simulink model "Respiratory"  (Simulink 6.4)
settings: Solver=ode45  StartTime=0.0  StopTime=10.0  RelTol=1e-3
values from neighbouring files (symbols this model uses):
  a1 = 0.3836    [Dissociation_Spencer_IC.m]    (also in Gas_Exchange_IC.m; Respiratory_IC.m)
  a2 = 1.819    [Dissociation_Spencer_IC.m]    (also in Gas_Exchange_IC.m; Respiratory_IC.m)
  alpha1 = 0.02598    [Dissociation_Spencer_IC.m]    (also in Gas_Exchange_IC.m; Respiratory_IC.m)
  alpha2 = 0.05591    [Dissociation_Spencer_IC.m]    (also in Gas_Exchange_IC.m; Respiratory_IC.m)
  beta1 = 0.012275    [Dissociation_Spencer_IC.m]    (also in Gas_Exchange_IC.m; Respiratory_IC.m)
  beta2 = 0.03255    [Dissociation_Spencer_IC.m]    (also in Gas_Exchange_IC.m; Respiratory_IC.m)
  C1 = 9    [Dissociation_Spencer_IC.m]    (also in Gas_Exchange_IC.m; Respiratory_IC.m)
  C2 = 87.00    (= 87)    [Dissociation_Spencer_IC.m]    (also in Gas_Exchange_IC.m; Respiratory_IC.m)
  Circadian_Period = 24    [Respiratory_IC.m]    (also in State_UA_Khoo_IC.m)
  CvCO2IC = 0.5116    [Body_Khoo_IC.m]    (also in Gas_Exchange_IC.m; Respiratory_IC.m = 0.5247)
  CvO2IC = 0.1672    [Body_Khoo_IC.m]    (also in Gas_Exchange_IC.m; Respiratory_IC.m = 0.1639)
  Dead1CO2IC = 0.1020    (= 0.102)    [Dead_Space_Khoo_IC.m]    (also in Gas_Exchange_IC.m; Respiratory_IC.m = 39.5616)
  Dead1O2IC = 149.8824    [Dead_Space_Khoo_IC.m]    (also in Gas_Exchange_IC.m; Respiratory_IC.m = 104.3637)
  Dead2CO2IC = 0.5274    [Dead_Space_Khoo_IC.m]    (also in Gas_Exchange_IC.m; Respiratory_IC.m = 39.6736)
  Dead2O2IC = 149.3923    [Dead_Space_Khoo_IC.m]    (also in Gas_Exchange_IC.m; Respiratory_IC.m = 104.2258)
  Dead3CO2IC = 2.2996    [Dead_Space_Khoo_IC.m]    (also in Gas_Exchange_IC.m; Respiratory_IC.m = 39.8127)
  Dead3O2IC = 147.3503    [Dead_Space_Khoo_IC.m]    (also in Gas_Exchange_IC.m; Respiratory_IC.m = 104.0505)
  Dead4CO2IC = 8.2293    [Dead_Space_Khoo_IC.m]    (also in Gas_Exchange_IC.m; Respiratory_IC.m = 40.0061)
  Dead4O2IC = 140.5179    [Dead_Space_Khoo_IC.m]    (also in Gas_Exchange_IC.m; Respiratory_IC.m = 103.8005)
  Dead5CO2IC = 22.0757    [Dead_Space_Khoo_IC.m]    (also in Gas_Exchange_IC.m; Respiratory_IC.m = 40.3359)
  Dead5O2IC = 124.5641    [Dead_Space_Khoo_IC.m]    (also in Gas_Exchange_IC.m; Respiratory_IC.m = 103.3579)
  E_CW = 5    [Pleural_Schuessler_IC.m]    (also in Pmus_Flow_Younes_IC.m; Resp_Mech_IC.m; Respiratory_IC.m)
  E_L = 5    [Pleural_Schuessler_IC.m]    (also in Pmus_Flow_Younes_IC.m; Resp_Mech_IC.m; Respiratory_IC.m)
  fc = 0.4/60    (= 0.00666666666667)    [Respiratory_IC.m]    (also in State_UA_Khoo_IC.m)
  FlowIC = 0    [Pmus_Flow_Younes_IC.m]    (also in Resp_Mech_IC.m; Respiratory_IC.m)
  gc = 0.008/60    (= 0.000133333333333)    [Respiratory_IC.m]    (also in State_UA_Khoo_IC.m)
  h = 0.0183    [Brain_Khoo_IC.m]    (also in Gas_Exchange_IC.m; Respiratory_IC.m)
  K1 = 13    [Dissociation_Spencer_IC.m]    (also in Gas_Exchange_IC.m; Respiratory_IC.m)
  K2 = 194.4    [Dissociation_Spencer_IC.m]    (also in Gas_Exchange_IC.m; Respiratory_IC.m)
  MRbCO2 = 0.0517    [Brain_Khoo_IC.m]    (also in Gas_Exchange_IC.m; Respiratory_IC.m)
  MRCO2 = 0.0033    [Body_Khoo_IC.m]    (also in Gas_Exchange_IC.m; Respiratory_IC.m)
  MRO2 = 0.0038    [Body_Khoo_IC.m]    (also in Gas_Exchange_IC.m; Respiratory_IC.m)
  PACO2_delayIC = 39.6041    [Cardio_Mix_Lange_IC.m]    (also in Gas_Exchange_IC.m; Respiratory_IC.m = 40.4448)
  PaCO2firstIC = 0.2150    (= 0.215)    [Cardio_Mix_Lange_IC.m]    (also in Gas_Exchange_IC.m; Respiratory_IC.m = -0.2465)
  PACO2IC = 37.1484    [Gas_Exchange_IC.m]    (also in Lungs_Khoo_IC.m; Respiratory_IC.m = 40.9432)
  PaCO2secondIC = 38.4577    [Cardio_Mix_Lange_IC.m]    (also in Gas_Exchange_IC.m; Respiratory_IC.m = 40.3928)
  PAO2_delayIC = 103.8436    [Cardio_Mix_Lange_IC.m]    (also in Gas_Exchange_IC.m; Respiratory_IC.m = 103.1223)
  PaO2firstIC = -0.2838    [Cardio_Mix_Lange_IC.m]    (also in Gas_Exchange_IC.m; Respiratory_IC.m = 0.3557)
  PAO2IC = 107.1983    [Gas_Exchange_IC.m]    (also in Lungs_Khoo_IC.m; Respiratory_IC.m = 102.5153)
  PaO2secondIC = 105.4828    [Cardio_Mix_Lange_IC.m]    (also in Gas_Exchange_IC.m; Respiratory_IC.m = 103.1435)
  PbCO2IC = 48.2858    [Brain_Khoo_IC.m]    (also in Gas_Exchange_IC.m; Respiratory_IC.m = 48.5383)
  PICO2 = 0    [Dead_Space_Khoo_IC.m]    (also in Gas_Exchange_IC.m; Respiratory_IC.m)
  PICO2_change = 0    [Respiratory_IC.m]
  PIO2 = 150    [Dead_Space_Khoo_IC.m]    (also in Gas_Exchange_IC.m; Respiratory_IC.m)
  PIO2_change = -90    [Mech_vent_test.m]    (also in Respiratory_IC.m = 0)
  Pt_frcIC1 = 0    [Pmus_Flow_Younes_IC.m]    (also in Resp_Mech_IC.m; Respiratory_IC.m)
  Pt_frcIC2 = 0    [Pmus_Flow_Younes_IC.m]    (also in Resp_Mech_IC.m; Respiratory_IC.m)
  QdBo = 0.8333    [Brain_Khoo_IC.m]    (also in Gas_Exchange_IC.m; Respiratory_IC.m)
  R_AW = 1.27    [Pleural_Schuessler_IC.m]    (also in Pmus_Flow_Younes_IC.m; Resp_Mech_IC.m; Respiratory_IC.m)
  R_CW = 1.03    [Pleural_Schuessler_IC.m]    (also in Pmus_Flow_Younes_IC.m; Resp_Mech_IC.m; Respiratory_IC.m)
  R_L = 1.69    [Pleural_Schuessler_IC.m]    (also in Pmus_Flow_Younes_IC.m; Resp_Mech_IC.m; Respiratory_IC.m)
  RC = 0.06    [Pleural_Schuessler_IC.m]    (also in Pmus_Flow_Younes_IC.m; Resp_Mech_IC.m; Respiratory_IC.m)
  rc = 0.2/60    (= 0.00333333333333)    [Respiratory_IC.m]    (also in State_UA_Khoo_IC.m)
  SbCO2 = 0.3600    (= 0.36)    [Brain_Khoo_IC.m]    (also in Gas_Exchange_IC.m; Respiratory_IC.m)
  SCO2 = 0.0043    [Brain_Khoo_IC.m]    (also in Gas_Exchange_IC.m; Respiratory_IC.m)
  SWAo = 0.007    [Respiratory_IC.m]    (also in State_UA_Khoo_IC.m)
  T1 = 1    [Cardio_Mix_Lange_IC.m]    (also in Gas_Exchange_IC.m; Respiratory_IC.m)
  T2 = 2    [Cardio_Mix_Lange_IC.m]    (also in Gas_Exchange_IC.m; Respiratory_IC.m)
  t_CO2_duration = 0    [Respiratory_IC.m]
  t_CO2_start = 0    [Respiratory_IC.m]
  t_end_UA = 0    [Respiratory_IC.m]    (also in State_UA_Khoo_IC.m)
  t_O2_duration = 0    [Mech_vent_test.m]    (also in Respiratory_IC.m)
  t_O2_start = 0    [Mech_vent_test.m]    (also in Respiratory_IC.m)
  t_start_UA = 0    [Respiratory_IC.m]    (also in State_UA_Khoo_IC.m)
  time_step = time_step    [acquire_data.m]    (also in acquire_data_save.m)
  VC = 5    [Pmus_Flow_Younes_IC.m]    (also in Resp_Mech_IC.m; Respiratory_IC.m)
  Vdead1 = 0.03    [Dead_Space_Khoo_IC.m]    (also in Gas_Exchange_IC.m; Respiratory_IC.m)
  Vdead2 = 0.03    [Dead_Space_Khoo_IC.m]    (also in Gas_Exchange_IC.m; Respiratory_IC.m)
  Vdead3 = 0.03    [Dead_Space_Khoo_IC.m]    (also in Gas_Exchange_IC.m; Respiratory_IC.m)
  Vdead4 = 0.03    [Dead_Space_Khoo_IC.m]    (also in Gas_Exchange_IC.m; Respiratory_IC.m)
  Vdead5 = 0.03    [Dead_Space_Khoo_IC.m]    (also in Gas_Exchange_IC.m; Respiratory_IC.m)
  VTCO2 = 15    [Body_Khoo_IC.m]    (also in Gas_Exchange_IC.m; Respiratory_IC.m)
  VtIC = 0    [Pmus_Flow_Younes_IC.m]    (also in Resp_Mech_IC.m; Respiratory_IC.m)
  VTO2 = 6    [Body_Khoo_IC.m]    (also in Gas_Exchange_IC.m; Respiratory_IC.m)
  Z = 0.0227    [Dissociation_Spencer_IC.m]    (also in Gas_Exchange_IC.m; Respiratory_IC.m)
undefined symbols (not defined in the file or in its folder): A_0_ua, Arousal_UAIC, b_ua, C_ua_awake, DAY, K_ua, R_LAW, R_trachea
libraries: simulink x1, simulink_extras x1
(part 2 of 2)

== system Respiratory/Gas Exchange/GAS EXCHANGE IN THE LUNGS/CO2 Gas Exchange in the Lungs ==
  CaCO2 : Inport
  CVCO2 : Inport  Port=2
  Pd5CO2 : Inport  Port=3
  Vt - Tidal Volume : Inport  Port=4
  Flow : Inport  Port=5
  "Q " : Inport  Port=6
  Fcn -11 blocks : Fcn  Expr=(((u(2) >=0) * u(2) * u(1) + (u(2) <0) * 0 ) + (u(3) - u(4)) *u(5) * ( lambda*(1-s) ) )/( u(6)+VLCO2 )
  Integrator : Integrator  InitialCondition=PACO2IC
  Mux : Mux  Inputs=6
  sum1 : Sum  Inputs=-+  SaturateOnIntegerOverflow=on  InputSameDT=on
  PACO2 : Outport
  tag scope: PACO2IC=global
  wires:
  "Q "/1 -> Mux/5
  CVCO2/1 -> Mux/3
  CaCO2/1 -> Mux/4
  Fcn -11 blocks/1 -> Integrator/1
  Integrator/1 -> [PACO2IC], PACO2/1, sum1/1
  Pd5CO2/1 -> sum1/2
  Mux/1 -> Fcn -11 blocks/1
  sum1/1 -> Mux/1
  Flow/1 -> Mux/2
  Vt - Tidal Volume/1 -> Mux/6

== system Respiratory/Gas Exchange/GAS EXCHANGE IN THE LUNGS/O2 Gas Exchange in the Lungs ==
  Vt - Tidal Volume : Inport
  Flow : Inport  Port=2
  Q : Inport  Port=3
  CaO2 : Inport  Port=4
  CVO2 : Inport  Port=5
  Pd5O2 : Inport  Port=6
  Fcn -11 blocks : Fcn  Expr=(((u(2) >=0) * u(2) * u(1) + (u(2) <0) * 0 ) + (u(4) - u(5)) *u(3) * ( lambda*(1-s) ) )/( u(6)+VLO2 )
  Integrator : Integrator  InitialCondition=PAO2IC  LimitOutput=on  LowerSaturationLimit=0
  Mux : Mux  Inputs=6
  Sum2 : Sum  Inputs=-+  SaturateOnIntegerOverflow=on  InputSameDT=on
  PAO2 : Outport
  tag scope: PAO2IC=global
  wires:
  Integrator/1 -> PAO2/1, [PAO2IC], Sum2/1
  Fcn -11 blocks/1 -> Integrator/1
  Pd5O2/1 -> Sum2/2
  Mux/1 -> Fcn -11 blocks/1
  Sum2/1 -> Mux/1
  Flow/1 -> Mux/2
  Q/1 -> Mux/3
  CVO2/1 -> Mux/4
  CaO2/1 -> Mux/5
  Vt - Tidal Volume/1 -> Mux/6

== system Respiratory/Respiratory_Mechanics/Pleural_Pressure1/Pa ==
  "Flow   " : Inport
  "Pao " : Inport  Port=2
  Fcn : Fcn  Expr=(u>=0)*u * (kaw1 + abs( (u>=0)*u) *kaw2)
  Fcn1 : Fcn  Expr=(u>=0)*u
  Sum2 : Sum  Inputs=+-  SaturateOnIntegerOverflow=on  InputSameDT=on
  "Pa " : Outport
  wires:
  "Flow   "/1 -> Fcn/1
  "Pao "/1 -> Sum2/1
  Sum2/1 -> Fcn1/1
  Fcn/1 -> Sum2/2
  Fcn1/1 -> "Pa "/1

== system Respiratory/Respiratory_Mechanics/Pleural_Pressure1/Pcw ==
  Vt : Inport
  Flow : Inport  Port=2
  Fcn : Fcn  Expr=(u>=0)*u
  Pcw_0 : Constant  Value=-1  OutDataType=sfix(16)  ConRadixGroup=Use specified scaling  OutScaling=2^0  SampleTime=inf  FramePeriod=inf
  Product3 : Product  SaturateOnIntegerOverflow=on  InputSameDT=on
  Product4 : Product  SaturateOnIntegerOverflow=on  InputSameDT=on
  Sum3 : Sum  Inputs=+++  SaturateOnIntegerOverflow=on  InputSameDT=on
  elastance : Constant  Value=E_CW  OutDataType=sfix(16)  ConRadixGroup=Use specified scaling  OutScaling=2^0  SampleTime=inf  FramePeriod=inf
  "resistance " : Constant  Value=R_CW  OutDataType=sfix(16)  ConRadixGroup=Use specified scaling  OutScaling=2^0  SampleTime=inf  FramePeriod=inf
  "Pcw  " : Outport
  wires:
  Fcn/1 -> Product3/2
  Vt/1 -> Product4/1
  elastance/1 -> Product4/2
  Sum3/1 -> "Pcw  "/1
  Product4/1 -> Sum3/2
  Flow/1 -> Fcn/1
  Product3/1 -> Sum3/1
  "resistance "/1 -> Product3/1
  Pcw_0/1 -> Sum3/3

== system Respiratory/Respiratory_Mechanics/Respiratory Muscles Activity1/Resp Muscle Reaction ==
  RespMus Drive : Inport
  Step Size : Inport  Port=2
  0.735539 : Gain
  Fcn : Fcn  Expr=u(1) + u(2) + (u(2) *u(5)/u(4) - u(3)+u(1)) * (exp(-u(4)/u(5)) - 1)
  Memory : Memory  X0=Pt_frcIC1  InheritSampleTime=on
  Memory1 : Memory  Orientation=left  X0=Pt_frcIC2  InheritSampleTime=on  LinearizeMemory=on
  Mux : Mux  Inputs=5
  RC1 : Constant  Value=RC  OutDataType=sfix(16)  ConRadixGroup=Use specified scaling  OutScaling=2^0  SampleTime=inf  FramePeriod=inf
  Sum4 : Sum  Inputs=+-  SaturateOnIntegerOverflow=on  InputSameDT=on
  Pt_frc : Outport
  wires:
  RespMus Drive/1 -> Sum4/1, Memory/1
  Sum4/1 -> Mux/2
  RC1/1 -> Mux/5
  Step Size/1 -> Mux/4
  Memory1/1 -> Mux/1
  Memory/1 -> Sum4/2, Mux/3
  Mux/1 -> Fcn/1
  Fcn/1 -> 0.735539/1
  0.735539/1 -> Pt_frc/1, Memory1/1

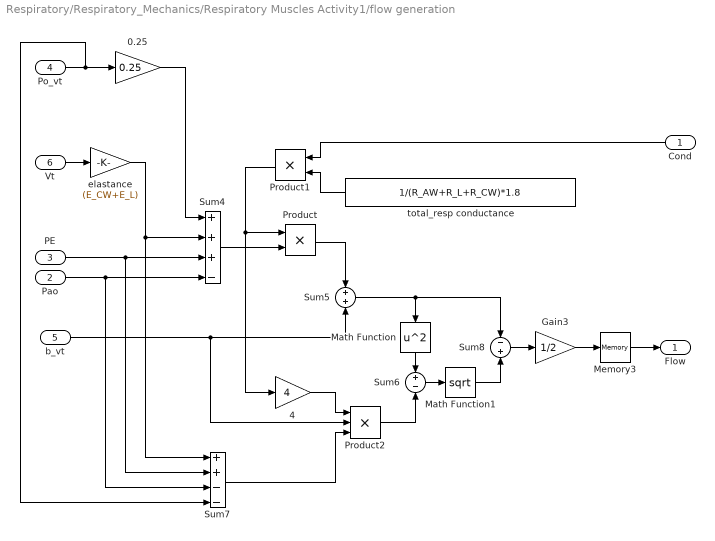
== system Respiratory/Respiratory_Mechanics/Respiratory Muscles Activity1/flow generation ==
  "Cond " : Inport  Orientation=left
  "Pao " : Inport  Port=2
  PE : Inport  Port=3
  "Po_vt " : Inport  Port=4
  b_vt : Inport  Port=5
  Vt : Inport  Port=6
  0.25 : Gain  Gain=0.25  SaturateOnIntegerOverflow=on
  4 : Gain  Gain=4  SaturateOnIntegerOverflow=on
  Gain3 : Gain  Gain=1/2  SaturateOnIntegerOverflow=on
  Math Function : Math  Orientation=down  Operator=square  SaturateOnIntegerOverflow=on
  Math Function1 : Math  Operator=sqrt  SaturateOnIntegerOverflow=on
  Memory3 : Memory  X0=FlowIC  InheritSampleTime=on
  Product : Product  SaturateOnIntegerOverflow=on  InputSameDT=on
  Product1 : Product  Orientation=left  SaturateOnIntegerOverflow=on  InputSameDT=on
  Product2 : Product  Inputs=3  SaturateOnIntegerOverflow=on  InputSameDT=on
  Sum4 : Sum  Inputs=+++-  SaturateOnIntegerOverflow=on  InputSameDT=on
  Sum5 : Sum  SaturateOnIntegerOverflow=on  InputSameDT=on
  Sum6 : Sum  Inputs=+-  SaturateOnIntegerOverflow=on  InputSameDT=on
  Sum7 : Sum  Inputs=++--  SaturateOnIntegerOverflow=on  InputSameDT=on
  Sum8 : Sum  Inputs=-+  SaturateOnIntegerOverflow=on  InputSameDT=on
  elastance : Gain  Gain=(E_CW+E_L)  SaturateOnIntegerOverflow=on
  total_resp conductance : Constant  Orientation=left  Value=1/(R_AW+R_L+R_CW)*1.8  OutDataType=sfix(16)  ConRadixGroup=Use specified scaling  OutScaling=2^0  SampleTime=inf  FramePeriod=inf
  Flow : Outport
  wires:
  0.25/1 -> Sum4/1
  total_resp conductance/1 -> Product1/2
  "Cond "/1 -> Product1/1
  Product1/1 -> 4/1, Product/1
  Gain3/1 -> Memory3/1
  Sum8/1 -> Gain3/1
  Sum5/1 -> Sum8/1, Math Function/1
  Math Function1/1 -> Sum8/2
  Sum6/1 -> Math Function1/1
  Product2/1 -> Sum6/2
  "Po_vt "/1 -> Sum7/4, 0.25/1
  "Pao "/1 -> Sum7/3, Sum4/4
  PE/1 -> Sum7/2, Sum4/3
  elastance/1 -> Sum7/1, Sum4/2
  Sum7/1 -> Product2/3
  b_vt/1 -> Product2/2, Sum5/2
  4/1 -> Product2/1
  Math Function/1 -> Sum6/1
  Product/1 -> Sum5/1
  Sum4/1 -> Product/2
  Vt/1 -> elastance/1
  Memory3/1 -> Flow/1

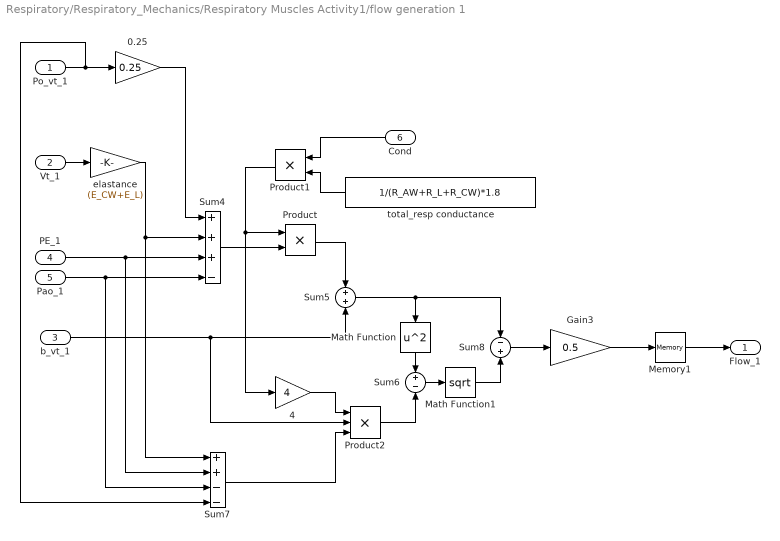
== system Respiratory/Respiratory_Mechanics/Respiratory Muscles Activity1/flow generation 1 ==
  Po_vt_1 : Inport
  Vt_1 : Inport  Port=2
  b_vt_1 : Inport  Port=3
  PE_1 : Inport  Port=4
  Pao_1 : Inport  Port=5
  "Cond " : Inport  Orientation=left  Port=6
  0.25 : Gain  Gain=0.25  SaturateOnIntegerOverflow=on
  4 : Gain  Gain=4  SaturateOnIntegerOverflow=on
  Gain3 : Gain  Gain=0.5  SaturateOnIntegerOverflow=on
  Math Function : Math  Orientation=down  Operator=square  SaturateOnIntegerOverflow=on
  Math Function1 : Math  Operator=sqrt  SaturateOnIntegerOverflow=on
  Memory1 : Memory  X0=FlowIC  InheritSampleTime=on
  Product : Product  SaturateOnIntegerOverflow=on  InputSameDT=on
  Product1 : Product  Orientation=left  SaturateOnIntegerOverflow=on  InputSameDT=on
  Product2 : Product  Inputs=3  SaturateOnIntegerOverflow=on  InputSameDT=on
  Sum4 : Sum  Inputs=+++-  SaturateOnIntegerOverflow=on  InputSameDT=on
  Sum5 : Sum  SaturateOnIntegerOverflow=on  InputSameDT=on
  Sum6 : Sum  Inputs=+-  SaturateOnIntegerOverflow=on  InputSameDT=on
  Sum7 : Sum  Inputs=++--  SaturateOnIntegerOverflow=on  InputSameDT=on
  Sum8 : Sum  Inputs=-+  SaturateOnIntegerOverflow=on  InputSameDT=on
  elastance : Gain  Gain=(E_CW+E_L)  SaturateOnIntegerOverflow=on
  total_resp conductance : Constant  Orientation=left  Value=1/(R_AW+R_L+R_CW)*1.8  OutDataType=sfix(16)  ConRadixGroup=Use specified scaling  OutScaling=2^0  SampleTime=inf  FramePeriod=inf
  Flow_1 : Outport
  wires:
  Vt_1/1 -> elastance/1
  Sum4/1 -> Product/2
  Product/1 -> Sum5/1
  Math Function/1 -> Sum6/1
  4/1 -> Product2/1
  b_vt_1/1 -> Sum5/2, Product2/2
  Sum7/1 -> Product2/3
  elastance/1 -> Sum4/2, Sum7/1
  PE_1/1 -> Sum4/3, Sum7/2
  Pao_1/1 -> Sum4/4, Sum7/3
  Po_vt_1/1 -> 0.25/1, Sum7/4
  Product2/1 -> Sum6/2
  Sum6/1 -> Math Function1/1
  Math Function1/1 -> Sum8/2
  Sum5/1 -> Math Function/1, Sum8/1
  Sum8/1 -> Gain3/1
  Gain3/1 -> Memory1/1
  Product1/1 -> Product/1, 4/1
  "Cond "/1 -> Product1/1
  total_resp conductance/1 -> Product1/2
  0.25/1 -> Sum4/1
  Memory1/1 -> Flow_1/1

== system Respiratory/Sleep Mechanism/Saving CircadianProcess/Switch Case Action Subsystem ==
  In1 : Inport
  Action Port : ActionPort
  To File : ToFile  Filename=CircadianProcess1.mat  MatrixName=H_L_CircardianLow_RBM_SWA  SampleTime=sampletime
  wires:
  In1/1 -> To File/1

== system Respiratory/Sleep Mechanism/Saving CircadianProcess/Switch Case Action Subsystem1 ==
  In1 : Inport
  Action Port : ActionPort
  To File : ToFile  Filename=CircadianProcess2.mat  MatrixName=H_L_CircardianLow_RBM_SWA  SampleTime=sampletime
  wires:
  In1/1 -> To File/1

== system Respiratory/Sleep Mechanism/Saving CircadianProcess/Switch Case Action Subsystem2 ==
  In1 : Inport
  Action Port : ActionPort
  To File : ToFile  Filename=CircadianProcess3.mat  MatrixName=H_L_CircardianLow_RBM_SWA  SampleTime=sampletime
  wires:
  In1/1 -> To File/1

== system Respiratory/Sleep Mechanism/Saving CircadianProcess/Switch Case Action Subsystem3 ==
  In1 : Inport
  Action Port : ActionPort
  To File : ToFile  Filename=CircadianProcess10.mat  MatrixName=H_L_CircardianLow_RBM_SWA  SampleTime=sampletime
  wires:
  In1/1 -> To File/1

== system Respiratory/Sleep Mechanism/Saving CircadianProcess/Switch Case Action Subsystem4 ==
  In1 : Inport
  Action Port : ActionPort
  To File : ToFile  Filename=CircadianProcess4.mat  MatrixName=H_L_CircardianLow_RBM_SWA  SampleTime=sampletime
  wires:
  In1/1 -> To File/1

== system Respiratory/Sleep Mechanism/Saving CircadianProcess/Switch Case Action Subsystem5 ==
  In1 : Inport
  Action Port : ActionPort
  To File : ToFile  Filename=CircadianProcess5.mat  MatrixName=H_L_CircardianLow_RBM_SWA  SampleTime=sampletime
  wires:
  In1/1 -> To File/1

== system Respiratory/Sleep Mechanism/Saving CircadianProcess/Switch Case Action Subsystem6 ==
  In1 : Inport
  Action Port : ActionPort
  To File : ToFile  Filename=CircadianProcess6.mat  MatrixName=H_L_CircardianLow_RBM_SWA  SampleTime=sampletime
  wires:
  In1/1 -> To File/1

== system Respiratory/Sleep Mechanism/Saving CircadianProcess/Switch Case Action Subsystem7 ==
  In1 : Inport
  Action Port : ActionPort
  To File : ToFile  Filename=CircadianProcess7.mat  MatrixName=H_L_CircardianLow_RBM_SWA  SampleTime=sampletime
  wires:
  In1/1 -> To File/1

== system Respiratory/Sleep Mechanism/Saving CircadianProcess/Switch Case Action Subsystem8 ==
  In1 : Inport
  Action Port : ActionPort
  To File : ToFile  Filename=CircadianProcess8.mat  MatrixName=H_L_CircardianLow_RBM_SWA  SampleTime=sampletime
  wires:
  In1/1 -> To File/1

== system Respiratory/Sleep Mechanism/Saving CircadianProcess/Switch Case Action Subsystem9 ==
  In1 : Inport
  Action Port : ActionPort
  To File : ToFile  Filename=CircadianProcess9.mat  MatrixName=H_L_CircardianLow_RBM_SWA  SampleTime=sampletime
  wires:
  In1/1 -> To File/1

== system Respiratory/Upper_Airway_Mechanism/Upper_Airway_Model/ Flow in Upper Airway ==
  C_ua Upper Airway Compliance : Inport  Orientation=down
  P_ua Pressure in Upper Airways : Inport  Port=2
  Coefficient1 : Gain  Gain=-1  SaturateOnIntegerOverflow=on
  Coefficient2 : Gain  SaturateOnIntegerOverflow=on
  Constant : Constant  Value=R_trachea*10  OutDataType=sfix(16)  ConRadixGroup=Use specified scaling  OutScaling=2^0  SampleTime=inf  FramePeriod=inf
  Integrator : Integrator  Orientation=left  LimitOutput=on  UpperSaturationLimit=100  LowerSaturationLimit=-100
  Math Function : Math  Operator=reciprocal  SaturateOnIntegerOverflow=on
  Math Function1 : Math  Orientation=down  Operator=reciprocal  SaturateOnIntegerOverflow=on
  Memory : Memory
  Product : Product  Orientation=left  SaturateOnIntegerOverflow=on
  Product1 : Product  SaturateOnIntegerOverflow=on
  Sum : Sum  Inputs=|++  SaturateOnIntegerOverflow=on
  "Q_ua Upper Airway Flow " : Outport
  wires:
  Product1/1 -> Integrator/1, Memory/1
  P_ua Pressure in Upper Airways/1 -> Sum/1
  Sum/1 -> Product1/2
  C_ua Upper Airway Compliance/1 -> Math Function1/1
  Integrator/1 -> Product/1
  Product/1 -> Sum/2
  Constant/1 -> Math Function/1
  Math Function/1 -> Coefficient1/1
  Coefficient1/1 -> Product1/1
  Coefficient2/1 -> "Q_ua Upper Airway Flow "/1
  Memory/1 -> Coefficient2/1
  Math Function1/1 -> Product/2

== system Respiratory/Upper_Airway_Mechanism/Upper_Airway_Model/ Pressure in Upper Airway ==
  P_pl Pleural Pressure : Inport
  Q_la Lower Airway Flow : Inport  Port=2
  R_LA Lower Airways Resistance : Gain  Gain=R_LAW+R_L+R_CW  SaturateOnIntegerOverflow=on
  R_LA Lower Airways Resistance1 : Gain  Gain=0.7  SaturateOnIntegerOverflow=on
  Sum2 : Sum  SaturateOnIntegerOverflow=on
  "P_ua Upper Airway Pressure " : Outport  InitialOutput=[0]
  wires:
  Q_la Lower Airway Flow/1 -> R_LA Lower Airways Resistance/1  "Q_la Lower Airway Flow"
  P_pl Pleural Pressure/1 -> Sum2/2
  Sum2/1 -> "P_ua Upper Airway Pressure "/1
  R_LA Lower Airways Resistance/1 -> R_LA Lower Airways Resistance1/1
  R_LA Lower Airways Resistance1/1 -> Sum2/1

== system Respiratory/Upper_Airway_Mechanism/Upper_Airway_Model/Upper Airway Conductance3 ==
  C_ua_Upper_Airway_Compliance : Inport
  P_ua_Upper Airway Pressure : Inport  Port=2
  A_0_ua : Constant  Value=A_0_ua  OutDataType=sfix(16)  ConRadixGroup=Use specified scaling  OutScaling=2^0  SampleTime=inf  FramePeriod=inf
  Fcn : Fcn  Expr="( u(5) <=u(6) )* u(1)*0  + (u(5) >0.0)* u(1) * u(2) +  ( u(5) >u(6) )* (u(5) <=0.0) * ( u(7)>=0 ) * u(7)"
  Fcn1 : Fcn  Expr=u(2) * (1+u(3)*u(4)*u(5)) *u(1)
  Gain : Gain  Gain=-1  SaturateOnIntegerOverflow=on
  K_ua : Constant  Value=K_ua  OutDataType=sfix(16)  ConRadixGroup=Use specified scaling  OutScaling=2^0  SampleTime=inf  FramePeriod=inf
  Math Function : Math  Operator=reciprocal  SaturateOnIntegerOverflow=on
  Mux1 : Mux  Inputs=7
  Mux2 : Mux  Inputs=5
  Product : Product  SaturateOnIntegerOverflow=on
  Saturation : Saturate  UpperLimit=10  LowerLimit=-40
  b_ua : Constant  Value=b_ua*13  OutDataType=sfix(16)  ConRadixGroup=Use specified scaling  OutScaling=2^0  SampleTime=inf  FramePeriod=inf
  Y_ua_Upper Airway Conductance : Outport
  P_crit : Outport  Port=2
  wires:
  P_ua_Upper Airway Pressure/1 -> Mux1/5, Mux2/5  "P_ua"
  K_ua/1 -> Mux1/1, Mux2/1
  C_ua_Upper_Airway_Compliance/1 -> Mux1/4, Mux2/4, Product/1  "C_ua"
  b_ua/1 -> Mux1/3, Mux2/3, Product/2  "b_ua"
  A_0_ua/1 -> Mux1/2, Mux2/2  "A_0_ua"
  Mux1/1 -> Fcn/1
  Fcn/1 -> Y_ua_Upper Airway Conductance/1
  Fcn1/1 -> Mux1/7
  Mux2/1 -> Fcn1/1
  Gain/1 -> Saturation/1
  Product/1 -> Math Function/1
  Math Function/1 -> Gain/1
  Saturation/1 -> P_crit/1, Mux1/6

== system Respiratory/Upper_Airway_Mechanism/Upper_Airway_Model/Upper_Airway_Compliance ==
  "SI Sleep Wake State Index " : Inport
  Sleep/awake : Inport  Port=2
  % increase : Gain  Gain=35  SaturateOnIntegerOverflow=on
  Awake Upper Airway  Compliance : Constant  Value=C_ua_awake  OutDataType=sfix(16)  ConRadixGroup=Use specified scaling  OutScaling=2^0  SampleTime=inf  FramePeriod=inf
  Fcn : Fcn  Expr="( u(1) <=0 ) * u(2) + ( u(1) >=1) * u(2) * ( 1+u(3) ) +  ( u(1) >0 ) * ( u(1) <1 ) * u(2) * ( 1+u(3)*u(1)*u(1) * ( 1- u(4)))"
  Mux1 : Mux
  S_UA : Constant  Value=0.01  OutDataType=sfix(16)  ConRadixGroup=Use specified scaling  OutScaling=2^0  SampleTime=inf  FramePeriod=inf
  C_ua Upper Airway Compliance : Outport
  wires:
  Awake Upper Airway  Compliance/1 -> Mux1/2
  "SI Sleep Wake State Index "/1 -> Mux1/1
  % increase/1 -> Mux1/3
  Mux1/1 -> Fcn/1
  Fcn/1 -> C_ua Upper Airway Compliance/1
  S_UA/1 -> % increase/1
  Sleep/awake/1 -> Mux1/4

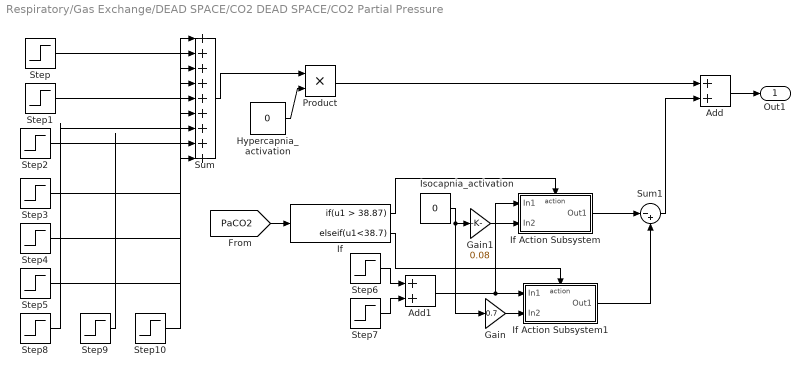
== system Respiratory/Gas Exchange/DEAD SPACE/CO2 DEAD SPACE/CO2 Partial Pressure ==
  Add : Sum  OutScaling=2^-10
  Add1 : Sum  OutScaling=2^-10
  Gain : Gain  Gain=0.7
  Gain1 : Gain  Gain=0.08
  Hypercapnia_activation : Constant  Value=0  OutDataType=sfix(16)  ConRadixGroup=Use specified scaling  OutScaling=2^0  SampleTime=inf  FramePeriod=inf
  If : If  IfExpression=u1 > 38.87  ElseIfExpressions=u1<38.7  ShowElse=off
  If Action Subsystem : Subsystem  TreatAsAtomicUnit=on
  If Action Subsystem1 : Subsystem  TreatAsAtomicUnit=on
  Isocapnia_activation : Constant  Value=0  OutDataType=sfix(16)  ConRadixGroup=Use specified scaling  OutScaling=2^0  SampleTime=inf  FramePeriod=inf
  Product : Product  RndMeth=Zero
  Step : Step  Time=begin_time  Before=init_value  After=final_value/8  SampleTime=0
  Step1 : Step  Time=end_time  After=init_value-final_value  SampleTime=0
  Step10 : Step  Time=begin_time+18  Before=init_value  After=final_value/8  SampleTime=0
  Step2 : Step  Time=begin_time+3  Before=init_value  After=final_value/8  SampleTime=0
  Step3 : Step  Time=begin_time+6  Before=init_value  After=final_value/8  SampleTime=0
  Step4 : Step  Time=begin_time+9  Before=init_value  After=final_value/8  SampleTime=0
  Step5 : Step  Time=begin_time+12  Before=init_value  After=final_value/8  SampleTime=0
  Step6 : Step  Time=begin_time  SampleTime=0
  Step7 : Step  Time=end_time  After=-1  SampleTime=0
  Step8 : Step  Time=begin_time+14  Before=init_value  After=final_value/8  SampleTime=0
  Step9 : Step  Time=begin_time+16  Before=init_value  After=final_value/8  SampleTime=0
  Sum : Sum  Inputs=|+++++++++  SaturateOnIntegerOverflow=on  InputSameDT=on
  Sum1 : Sum  Inputs=|-+
  Out1 : Outport
  wires:
  [PaCO2] -> If/1
  Add/1 -> Out1/1
  Step6/1 -> Add1/1
  Step7/1 -> Add1/2
  Sum1/1 -> Add/2
  If/1 -> If Action Subsystem/Action
  If/2 -> If Action Subsystem1/Action
  Add1/1 -> If Action Subsystem1/1(In1), If Action Subsystem/1(In1)
  Isocapnia_activation/1 -> Gain1/1, Gain/1
  If Action Subsystem/1(Out1) -> Sum1/1
  If Action Subsystem1/1(Out1) -> Sum1/2
  Step/1 -> Sum/1
  Step1/1 -> Sum/2
  Step2/1 -> Sum/3
  Step3/1 -> Sum/4
  Step4/1 -> Sum/5
  Step5/1 -> Sum/6
  Sum/1 -> Product/1
  Hypercapnia_activation/1 -> Product/2
  Product/1 -> Add/1
  Step8/1 -> Sum/7
  Step9/1 -> Sum/8
  Step10/1 -> Sum/9
  Gain/1 -> If Action Subsystem1/2(In2)
  Gain1/1 -> If Action Subsystem/2(In2)

== system Respiratory/Gas Exchange/DEAD SPACE/CO2 DEAD SPACE/Pd(1)CO2 ==
  PICO2 : Inport
  Flow : Inport  Port=2
  Pd(2)CO2 : Inport  Port=3
  1/Vdead1 : Gain  Gain=1/Vdead1  SaturateOnIntegerOverflow=on
  Abs (v.t) : Abs  SaturateOnIntegerOverflow=on  SampleTime=-1
  Integrator : Integrator  InitialCondition=Dead1CO2IC
  Product : Product  SaturateOnIntegerOverflow=on  InputSameDT=on
  Sum : Sum  Inputs=-+  SaturateOnIntegerOverflow=on  InputSameDT=on
  Switch : Switch  SaturateOnIntegerOverflow=on  InputSameDT=on
  Pd(1)CO2 : Outport
  tag scope: Dead1CO2IC=global
  wires:
  Flow/1 -> Abs (v.t)/1, Switch/2
  Abs (v.t)/1 -> Product/2
  Switch/1 -> Sum/2
  Product/1 -> 1/Vdead1/1
  1/Vdead1/1 -> Integrator/1
  Integrator/1 -> [Dead1CO2IC], Pd(1)CO2/1, Sum/1
  Sum/1 -> Product/1
  PICO2/1 -> Switch/1
  Pd(2)CO2/1 -> Switch/3

== system Respiratory/Gas Exchange/DEAD SPACE/CO2 DEAD SPACE/Pd(2)CO2 ==
  Pd(1)CO2 : Inport
  Flow : Inport  Port=2
  Pd(3)CO2 : Inport  Port=3
  1/Vdead2 : Gain  Gain=1/Vdead2  SaturateOnIntegerOverflow=on
  Abs (v.t) : Abs  SaturateOnIntegerOverflow=on  SampleTime=-1
  Integrator : Integrator  InitialCondition=Dead2CO2IC
  Product : Product  SaturateOnIntegerOverflow=on  InputSameDT=on
  Sum : Sum  Inputs=-+  SaturateOnIntegerOverflow=on  InputSameDT=on
  Switch : Switch  SaturateOnIntegerOverflow=on  InputSameDT=on
  Pd(2)CO2 : Outport
  tag scope: Dead2CO2IC=global
  wires:
  Integrator/1 -> Pd(2)CO2/1, Sum/1, [Dead2CO2IC]
  Abs (v.t)/1 -> Product/2
  Flow/1 -> Abs (v.t)/1, Switch/2
  Pd(3)CO2/1 -> Switch/3
  Pd(1)CO2/1 -> Switch/1
  Sum/1 -> Product/1
  1/Vdead2/1 -> Integrator/1
  Product/1 -> 1/Vdead2/1
  Switch/1 -> Sum/2

== system Respiratory/Gas Exchange/DEAD SPACE/CO2 DEAD SPACE/Pd(3)CO2 ==
  Pd(2)CO2 : Inport
  Flow : Inport  Port=2
  Pd(4)CO2 : Inport  Port=3
  1/Vdead3 : Gain  Gain=1/Vdead3  SaturateOnIntegerOverflow=on
  Abs (v.t) : Abs  SaturateOnIntegerOverflow=on  SampleTime=-1
  Integrator : Integrator  InitialCondition=Dead3CO2IC
  Product : Product  SaturateOnIntegerOverflow=on  InputSameDT=on
  Sum : Sum  Inputs=-+  SaturateOnIntegerOverflow=on  InputSameDT=on
  Switch : Switch  SaturateOnIntegerOverflow=on  InputSameDT=on
  Pd(3)CO2 : Outport
  tag scope: Dead3CO2IC=global
  wires:
  Abs (v.t)/1 -> Product/2
  Flow/1 -> Abs (v.t)/1, Switch/2
  Switch/1 -> Sum/2
  Product/1 -> 1/Vdead3/1
  1/Vdead3/1 -> Integrator/1
  Integrator/1 -> Sum/1, Pd(3)CO2/1, [Dead3CO2IC]
  Sum/1 -> Product/1
  Pd(2)CO2/1 -> Switch/1
  Pd(4)CO2/1 -> Switch/3

== system Respiratory/Gas Exchange/DEAD SPACE/CO2 DEAD SPACE/Pd(4)CO2 ==
  Pd(3)CO2 : Inport
  Flow : Inport  Port=2
  Pd(5)CO2 : Inport  Port=3
  1/Vdead4 : Gain  Gain=1/Vdead4  SaturateOnIntegerOverflow=on
  Abs (v.t) : Abs  SaturateOnIntegerOverflow=on  SampleTime=-1
  Integrator : Integrator  InitialCondition=Dead4CO2IC
  Product : Product  SaturateOnIntegerOverflow=on  InputSameDT=on
  Sum : Sum  Inputs=-+  SaturateOnIntegerOverflow=on  InputSameDT=on
  Switch : Switch  SaturateOnIntegerOverflow=on  InputSameDT=on
  Pd(4)CO2 : Outport
  tag scope: Dead4CO2IC=global
  wires:
  Abs (v.t)/1 -> Product/2
  Flow/1 -> Abs (v.t)/1, Switch/2
  Pd(5)CO2/1 -> Switch/3
  Pd(3)CO2/1 -> Switch/1
  Sum/1 -> Product/1
  1/Vdead4/1 -> Integrator/1
  Product/1 -> 1/Vdead4/1
  Switch/1 -> Sum/2
  Integrator/1 -> Pd(4)CO2/1, [Dead4CO2IC], Sum/1

== system Respiratory/Gas Exchange/DEAD SPACE/CO2 DEAD SPACE/Pd(5)CO2 ==
  Pd(4)CO2 : Inport
  Flow : Inport  Port=2
  PACO2 : Inport  Port=3
  1/Vdead5 : Gain  Gain=1/Vdead5  SaturateOnIntegerOverflow=on
  Abs (v.t) : Abs  SaturateOnIntegerOverflow=on  SampleTime=-1
  Integrator : Integrator  InitialCondition=Dead5CO2IC
  Product : Product  SaturateOnIntegerOverflow=on  InputSameDT=on
  Sum : Sum  Inputs=-+  SaturateOnIntegerOverflow=on  InputSameDT=on
  Switch : Switch  SaturateOnIntegerOverflow=on  InputSameDT=on
  Pd(5)CO2 : Outport
  tag scope: Dead5CO2IC=global
  wires:
  Abs (v.t)/1 -> Product/2
  Flow/1 -> Abs (v.t)/1, Switch/2
  Switch/1 -> Sum/2
  Product/1 -> 1/Vdead5/1
  1/Vdead5/1 -> Integrator/1
  Integrator/1 -> Sum/1, Pd(5)CO2/1, [Dead5CO2IC]
  Sum/1 -> Product/1
  Pd(4)CO2/1 -> Switch/1
  PACO2/1 -> Switch/3

== system Respiratory/Gas Exchange/DEAD SPACE/O2 DEAD SPACE/O2 Partial Pressure ==
  Step : Step  Time=begin_time  Before=init_value  After=final_value  SampleTime=0
  Step1 : Step  Time=end_time  After=init_value-final_value  SampleTime=0
  Sum : Sum  Inputs=|++  SaturateOnIntegerOverflow=on  InputSameDT=on
  Out1 : Outport
  wires:
  Sum/1 -> Out1/1
  Step1/1 -> Sum/2
  Step/1 -> Sum/1

== system Respiratory/Gas Exchange/DEAD SPACE/O2 DEAD SPACE/Pd(1)O2 ==
  PIO2 : Inport
  Flow : Inport  Port=2
  Pd(2)O2 : Inport  Port=3
  1/Vdead1 : Gain  Gain=1/Vdead1  SaturateOnIntegerOverflow=on
  Abs (v.t) : Abs  SaturateOnIntegerOverflow=on  SampleTime=-1
  Integrator : Integrator  InitialCondition=Dead1O2IC
  Product : Product  SaturateOnIntegerOverflow=on  InputSameDT=on
  Sum : Sum  Inputs=-+  SaturateOnIntegerOverflow=on  InputSameDT=on
  Switch : Switch  SaturateOnIntegerOverflow=on  InputSameDT=on
  Pd(1)O2 : Outport
  tag scope: Dead1O2IC=global
  wires:
  Switch/1 -> Sum/2
  Pd(2)O2/1 -> Switch/3
  PIO2/1 -> Switch/1
  Sum/1 -> Product/1
  Integrator/1 -> Sum/1, Pd(1)O2/1, [Dead1O2IC]
  1/Vdead1/1 -> Integrator/1
  Product/1 -> 1/Vdead1/1
  Flow/1 -> Abs (v.t)/1, Switch/2
  Abs (v.t)/1 -> Product/2

== system Respiratory/Gas Exchange/DEAD SPACE/O2 DEAD SPACE/Pd(2)O2 ==
  Pd(1)O2 : Inport
  Flow : Inport  Port=2
  Pd(3)O2 : Inport  Port=3
  1/Vdead2 : Gain  Gain=1/Vdead2  SaturateOnIntegerOverflow=on
  Abs (v.t) : Abs  SaturateOnIntegerOverflow=on  SampleTime=-1
  Integrator : Integrator  InitialCondition=Dead2O2IC
  Product : Product  SaturateOnIntegerOverflow=on  InputSameDT=on
  Sum : Sum  Inputs=-+  SaturateOnIntegerOverflow=on  InputSameDT=on
  Switch : Switch  SaturateOnIntegerOverflow=on  InputSameDT=on
  Pd(2)O2 : Outport
  tag scope: Dead2O2IC=global
  wires:
  Abs (v.t)/1 -> Product/2
  Flow/1 -> Abs (v.t)/1, Switch/2
  Product/1 -> 1/Vdead2/1
  Integrator/1 -> [Dead2O2IC], Sum/1, Pd(2)O2/1
  Sum/1 -> Product/1
  Pd(1)O2/1 -> Switch/1
  Pd(3)O2/1 -> Switch/3
  Switch/1 -> Sum/2
  1/Vdead2/1 -> Integrator/1

== system Respiratory/Gas Exchange/DEAD SPACE/O2 DEAD SPACE/Pd(3)O2 ==
  Pd(2)O2 : Inport
  Flow : Inport  Port=2
  Pd(4)O2 : Inport  Port=3
  1/Vdead3 : Gain  Gain=1/Vdead3  SaturateOnIntegerOverflow=on
  Abs (v.t) : Abs  SaturateOnIntegerOverflow=on  SampleTime=-1
  Integrator : Integrator  InitialCondition=Dead3O2IC
  Product : Product  SaturateOnIntegerOverflow=on  InputSameDT=on
  Sum : Sum  Inputs=-+  SaturateOnIntegerOverflow=on  InputSameDT=on
  Switch : Switch  SaturateOnIntegerOverflow=on  InputSameDT=on
  Pd(3)O2 : Outport
  tag scope: Dead3O2IC=global
  wires:
  Switch/1 -> Sum/2
  Pd(4)O2/1 -> Switch/3
  Pd(2)O2/1 -> Switch/1
  Sum/1 -> Product/1
  Integrator/1 -> [Dead3O2IC], Sum/1, Pd(3)O2/1
  Product/1 -> 1/Vdead3/1
  Flow/1 -> Abs (v.t)/1, Switch/2
  Abs (v.t)/1 -> Product/2
  1/Vdead3/1 -> Integrator/1

== system Respiratory/Gas Exchange/DEAD SPACE/O2 DEAD SPACE/Pd(4)O2 ==
  Pd(3)O2 : Inport
  Flow : Inport  Port=2
  Pd(5)O2 : Inport  Port=3
  1/Vdead4 : Gain  Gain=1/Vdead4  SaturateOnIntegerOverflow=on
  Abs (v.t) : Abs  SaturateOnIntegerOverflow=on  SampleTime=-1
  Integrator : Integrator  InitialCondition=Dead4O2IC
  Product : Product  SaturateOnIntegerOverflow=on  InputSameDT=on
  Sum : Sum  Inputs=-+  SaturateOnIntegerOverflow=on  InputSameDT=on
  Switch : Switch  SaturateOnIntegerOverflow=on  InputSameDT=on
  Pd(4)O2 : Outport
  tag scope: Dead4O2IC=global
  wires:
  Abs (v.t)/1 -> Product/2
  Flow/1 -> Abs (v.t)/1, Switch/2
  Product/1 -> 1/Vdead4/1
  Integrator/1 -> Sum/1, Pd(4)O2/1, [Dead4O2IC]
  Sum/1 -> Product/1
  Pd(3)O2/1 -> Switch/1
  Pd(5)O2/1 -> Switch/3
  Switch/1 -> Sum/2
  1/Vdead4/1 -> Integrator/1

== system Respiratory/Gas Exchange/DEAD SPACE/O2 DEAD SPACE/Pd(5)O2 ==
  Pd(4)O2 : Inport
  Flow : Inport  Port=2
  PAO2 : Inport  Port=3
  1/Vdead5 : Gain  Gain=1/Vdead5  SaturateOnIntegerOverflow=on
  Abs (v.t) : Abs  SaturateOnIntegerOverflow=on  SampleTime=-1
  Integrator : Integrator  InitialCondition=Dead5O2IC
  Product : Product  SaturateOnIntegerOverflow=on  InputSameDT=on
  Sum : Sum  Inputs=-+  SaturateOnIntegerOverflow=on  InputSameDT=on
  Switch : Switch  SaturateOnIntegerOverflow=on  InputSameDT=on
  Pd(5)O2 : Outport
  tag scope: Dead5O2IC=global
  wires:
  Switch/1 -> Sum/2
  PAO2/1 -> Switch/3
  Pd(4)O2/1 -> Switch/1
  Sum/1 -> Product/1
  Integrator/1 -> Pd(5)O2/1, [Dead5O2IC], Sum/1
  Product/1 -> 1/Vdead5/1
  Flow/1 -> Abs (v.t)/1, Switch/2
  Abs (v.t)/1 -> Product/2
  1/Vdead5/1 -> Integrator/1

== system Respiratory/Gas Exchange/DEAD SPACE/CO2 DEAD SPACE/CO2 Partial Pressure/If Action Subsystem ==
  In1 : Inport
  In2 : Inport  Port=2
  Action Port : ActionPort
  Integrator : Integrator
  Product1 : Product  RndMeth=Zero
  Out1 : Outport  InitialOutput=0
  wires:
  Product1/1 -> Integrator/1
  In2/1 -> Product1/2
  In1/1 -> Product1/1
  Integrator/1 -> Out1/1

== system Respiratory/Gas Exchange/DEAD SPACE/CO2 DEAD SPACE/CO2 Partial Pressure/If Action Subsystem1 ==
  In1 : Inport
  In2 : Inport  Port=2
  Action Port : ActionPort
  Integrator : Integrator
  Product1 : Product  RndMeth=Zero
  Out1 : Outport  InitialOutput=0
  wires:
  Product1/1 -> Integrator/1
  In2/1 -> Product1/2
  In1/1 -> Product1/1
  Integrator/1 -> Out1/1

== matlab function Sleep Mechanism/Embedded MATLAB Function1 ==
  data: t0 input inherited; u2 input inherited; y output inherited; t input inherited
function y = fcn(t0, u2, t)
% This block supports an embeddable subset of the MATLAB language.
% See the help menu for details. 

% day = floor(para/3600/24);
% t0 = 0;
% count = 0;
% while count <=day
% if u1>0.5 %sleep/awake state change
%     t0 = t
% end
if u2 <0.5 %sleep start %sleep/awake state change
    y=0;
else %u2 >0.5 %(awake state)
    if (t>= t0 + 0.5*3600+5) && (t <= t0 + 0.5*3600+15*60+5)   %Breakfast
        y=22/60;
    elseif (t>= t0 + 5.5*3600+5) && (t <= t0 + 5.5*3600+30*60+5)%Lunch
        y=30/60;
    elseif (t>= t0 + 12*3600+5) && (t <=t0 + 12*3600+45*60+5)%dinner
        y=24/60;
    else %NREMs
        y=0; 
    end

end

== matlab function Sleep Mechanism/Embedded MATLAB Function ==
  data: t0 input inherited; u2 input inherited; y output inherited; t input inherited
function y = fcn(t0, u2, t)
% This block supports an embeddable subset of the MATLAB language.
% See the help menu for details. 

% day = floor(para/3600/24);
% t0 = 0;
% count = 0;
% while count <=day
% if u1>0.5 %sleep/awake state change
%     t0 = t
% end
if u2 >0.5 %awake state %sleep/awake state change
    y=0;
else %u2 <0.5 %(sleep start)
    if (t>=t0 + 0.85*1.8*3600+5) && (t <=t0 + 1*1.8*3600+5)   %1st REM
        y=1;
    elseif (t>=t0 + (1+0.85)*1.8*3600+5) && (t <=t0 + 2*1.8*3600+5)%2nd REM
        y=1;
    elseif (t>=t0 + (2+0.85)*1.8*3600+5) && (t <=t0 + 3*1.8*3600+5)%3rd REM
        y=1;
    elseif (t>=t0 + (3+0.85)*1.8*3600+5) && (t <=t0 + 4*1.8*3600+5)%4 REM
        y=1;
    elseif (t>=t0 + (4+0.85)*1.8*3600+5) && (t <=t0 + 5*1.8*3600+5)%5 REM
        y=1;
    elseif (t>=t0 + (5+0.85)*1.8*3600+5) && (t <=t0 + 6*1.8*3600+5)%6 REM
        y=1;
    else %NREMs
        y=0; 
    end

end
